simulink model "Leo_discreto"  (R2021a)
settings: Solver=ode5  StartTime=0.0  StopTime=15  FixedStep=ts  RelTol=1e-3
values from neighbouring files (symbols this model uses):
  A = [0 0 0 1;0 1446.9 213.6 -57.9;0 1 0 0;0 -126.3 -12.8 5.1]    [1_DiseñoRegulador_Seguidor_Discreto.m]    (also in Control_Seguimiento_Integrador_MATLAB.m = [0,1,0,0;0,-0.221772837618740,0.450086090591265,-0.661704776; Controlador.m = [0 1 0 0;0 -6.109*10^(-08)   2.828*10^(-5)  -7.749*10^(-6);0; Leo_Controlador.m = [0,1,0,0;0,-18.1491205715699,-0.241940259070541,-0.001617883; funcmotor.m = [0 1 0 0;0 par(1) par(2) par(3);0 0 0 1;0 par(4) par(5) par()
  B = [0;-122.6;0;10.7]    [1_DiseñoRegulador_Seguidor_Discreto.m]    (also in Control_Seguimiento_Integrador_MATLAB.m = [0;1.02819574469726;0;2.93672730148517]; Controlador.m = [0;-2.126*10^(-8);0;-293]; Leo_Controlador.m = [0;3.24704785577389;0;142.313463961677]; funcmotor.m = [0;par(7);0;par(8)])
  C = [1 0 0 0]    [1_DiseñoRegulador_Seguidor_Discreto.m]    (also in Control_Seguimiento_Integrador_MATLAB.m = [0 0 1 0]; Controlador.m = [0 0 1 0]; Leo_Controlador.m = [1 0 0 0;0 1 0 0;0 0 1 0; 0 0 0 1]; funcmotor.m = [0 0 1 0;1 0 0 0])
  D = [0]    [1_DiseñoRegulador_Seguidor_Discreto.m]    (also in Control_Seguimiento_Integrador_MATLAB.m; Controlador.m; Leo_Controlador.m = [0;0;0;0]; funcmotor.m = zeros(2,1))
  g1 = K(1)    [Leo_Controlador.m]
  k1 = Ka(1)    [1_DiseñoRegulador_Seguidor_Discreto.m]    (also in Controlador.m = -2.8342e-06; Leo_Controlador.m = K(1))
  k2 = Ka(2)    [1_DiseñoRegulador_Seguidor_Discreto.m]    (also in Controlador.m = -1925900; Leo_Controlador.m = K(2))
  k3 = Ka(3)    [1_DiseñoRegulador_Seguidor_Discreto.m]    (also in Controlador.m = -18.7082; Leo_Controlador.m = K(3))
  k4 = Ka(4)    [1_DiseñoRegulador_Seguidor_Discreto.m]    (also in Controlador.m = -0.1767; Leo_Controlador.m = K(4))
  ts = 1/1000    (= 0.001)    [Leo_Controlador.m]
settings Model: Creator=Usuario  LastModifiedBy=Sinso

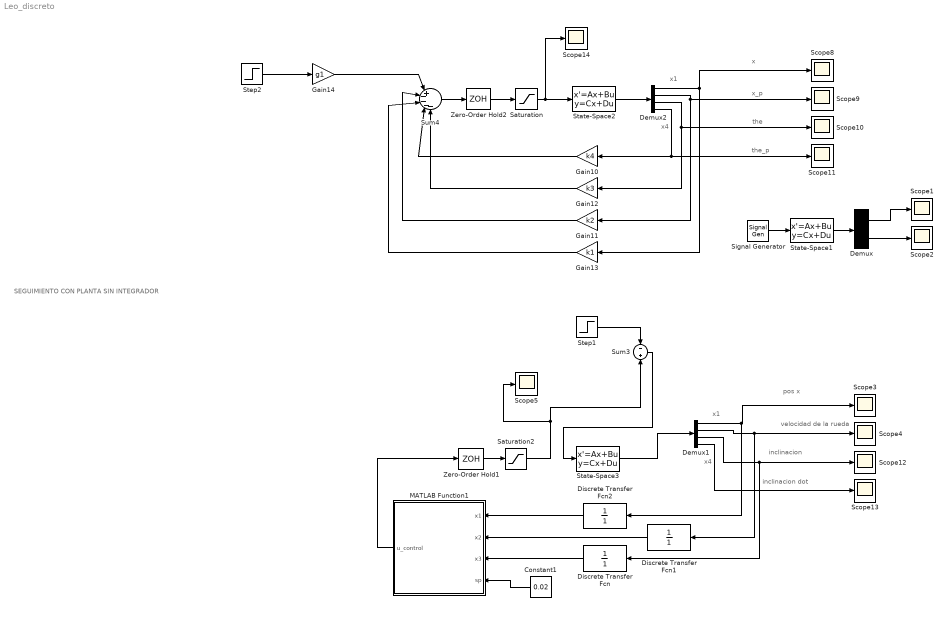
== system Leo_discreto ==
  note: x1
  note: x
  note: x_p
  note: x4
  note: the_p
  note: the
  note: inclinacion dot
  note: velocidad de la rueda
  note: x4
  note: x1
  note: SEGUIMIENTO CON PLANTA SIN INTEGRADOR
  note: pos x
  note: inclinacion
  Constant1 : Constant  Value=0.02
  Demux : Demux  Outputs=2
  Demux1 : Demux
  Demux2 : Demux
  Discrete Transfer Fcn : DiscreteTransferFcn  Denominator=[1]  SampleTime=ts
  Discrete Transfer Fcn1 : DiscreteTransferFcn  Denominator=[1]  SampleTime=ts
  Discrete Transfer Fcn2 : DiscreteTransferFcn  Denominator=[1]  SampleTime=ts
  Gain10 : Gain  Gain=k4
  Gain11 : Gain  Gain=k2
  Gain12 : Gain  Gain=k3
  Gain13 : Gain  Gain=k1
  Gain14 : Gain  Gain=g1
  MATLAB Function1 : MATLAB Function  TreatAsAtomicUnit=on  SystemSampleTime=ts
  Saturation : Saturate  UpperLimit=7.5  LowerLimit=-7.5
  Saturation2 : Saturate  UpperLimit=5  LowerLimit=-5
  Scope{1..5,8..14} (12 alike) : Scope
  Signal Generator : SignalGenerator  WaveForm=square  Amplitude=2.45  Frequency=10
  State-Space1 : StateSpace  A=A  B=B  C=C  D=D  InitialCondition=0
  State-Space2 : StateSpace  A=A  B=B  C=C  D=D  InitialCondition=0
  State-Space3 : StateSpace  A=A  B=B  C=C  D=D  InitialCondition=0  ParameterTunability=Optimized
  Step1 : Step  Time=2  After=0  SampleTime=0
  Step2 : Step  Time=0.1  After=0.02  SampleTime=0
  Sum3 : Sum  Inputs=-+
  Sum4 : Sum  Inputs=|+----
  Zero-Order Hold1 : ZeroOrderHold  SampleTime=ts
  Zero-Order Hold2 : ZeroOrderHold  SampleTime=ts
  wires:
  Step2/1 -> Gain14/1
  Gain14/1 -> Sum4/1
  State-Space2/1 -> Demux2/1
  Demux2/4 -> Scope11/1, Gain10/1
  Zero-Order Hold2/1 -> Saturation/1
  Gain10/1 -> Sum4/4
  Demux2/3 -> Gain12/1, Scope10/1
  Gain11/1 -> Sum4/2
  Sum4/1 -> Zero-Order Hold2/1
  Demux2/1 -> Gain13/1, Scope8/1
  Gain12/1 -> Sum4/5
  Gain13/1 -> Sum4/3
  Demux2/2 -> Scope9/1, Gain11/1
  Signal Generator/1 -> State-Space1/1
  State-Space1/1 -> Demux/1
  Demux/2 -> Scope2/1
  Demux/1 -> Scope1/1
  Saturation/1 -> Scope14/1, State-Space2/1
  Discrete Transfer Fcn2/1 -> MATLAB Function1/1(x1)
  Zero-Order Hold1/1 -> Saturation2/1
  Step1/1 -> Sum3/1
  Demux1/2 -> Discrete Transfer Fcn1/1, Scope4/1
  Constant1/1 -> MATLAB Function1/4(sp)
  Sum3/1 -> State-Space3/1
  Demux1/3 -> Scope12/1, Discrete Transfer Fcn/1
  State-Space3/1 -> Demux1/1
  Saturation2/1 -> Sum3/2, Scope5/1
  MATLAB Function1/1(u_control) -> Zero-Order Hold1/1
  Discrete Transfer Fcn1/1 -> MATLAB Function1/2(x2)
  Demux1/1 -> Discrete Transfer Fcn2/1, Scope3/1
  Discrete Transfer Fcn/1 -> MATLAB Function1/3(x3)
  Demux1/4 -> Scope13/1

== matlab function Leo_discreto/MATLAB Function1 ==
  settings: updateMethod=DISCRETE
  data: x1 input; u_control output; x2 input; x3 input; sp input
function u_control = fcn(x1,x2,x3,sp)
% a tss=1s
K=[1757.72666539153,-137.998491358980,-4.44560117253385,3.45586535840684]
% a tss=4s
% K=[6.86611978668566,0.374341451303578,-0.131544095753310,-0.0385560141760711]
% a tss=0.5s
% K=[2.812362664626447e+04,-3.553025131279486e+03,25.338419704681440,81.823397270692180]
% a tss=0.75s
% K=[5.555284275805325e+03,-5.805583908220522e+02,-4.821184541747814,13.703290059762757]
% a tss=2s y sobreimpulso
% K=[1.952016525488400e+02,-17.086879176997847,-0.046884032894643,0.416056059757730]

k1=K(1);
k2=K(2);
k3=K(3);
k4=K(4);
g1=k1;
T=0.001;

persistent x3_ant;

if isempty(x3_ant)
    x3_ant=0;
end

x4=(x3-x3_ant)/T;

u_control=g1*sp-(k1*x1+k2*x2+k3*x3+k4*x4);

x3_ant=x3;
